simulink model "register"  (R2024a)
settings: Solver=FixedStepDiscrete  StartTime=1  StopTime=inf  RelTol=1e-3  EnableMultiTasking=on
libraries: simulink_extras x5
settings Model: Creator=nunkesser  LastModifiedBy=nunkesser
settings SolverCC: AlgebraicLoopSolver=TrustRegion
settings DataIOCC: LimitDataPoints=on  SaveFormat=Array  ReturnWorkspaceOutputs=off
settings OptimizationCC: LifeSpan=inf
settings DebuggingCC: SolverPrmCheckMsg=warning  UnconnectedInputMsg=warning  UnconnectedOutputMsg=warning  UnconnectedLineMsg=warning  SFUnexpectedBacktrackingDiag=warning  SFNoUnconditionalDefaultTransitionDiag=warning  SFExecutionAtInitializationDiag=none  ArithmeticOperatorsInVariantConditions=warning
settings HardwareCC: ProdBitPerPointer=32  ProdBitPerSizeT=32  ProdBitPerPtrDiffT=32  ProdLargestAtomicFloat=None  ProdIntDivRoundTo=Undefined  ProdEndianess=Unspecified  ProdWordSize=32  ProdHWDeviceType=32-bit Generic
settings ModelReferenceCC: PropagateSignalLabelsOutOfModel=off
settings SFSimCC: SimUseLocalCustomCode=off  CustomCodeUndefinedFunction=UseInterfaceOnly
settings RTWCC: RTWUseLocalCustomCode=off  GPUComputeCapability=3.5
settings CodeAppCC: StateflowObjectComments=on
settings GRTTargetCC: TargetLangStandard=C89/C90 (ANSI)
settings ConfigComp: CovMetricSettings=dw  CovSaveCumulativeToWorkspaceVar=on  CovSaveSingleToWorkspaceVar=on  CovExternalEMLEnable=off  CovSFcnEnable=off
settings ConfigurationSet: Description=SimMechanics 2G

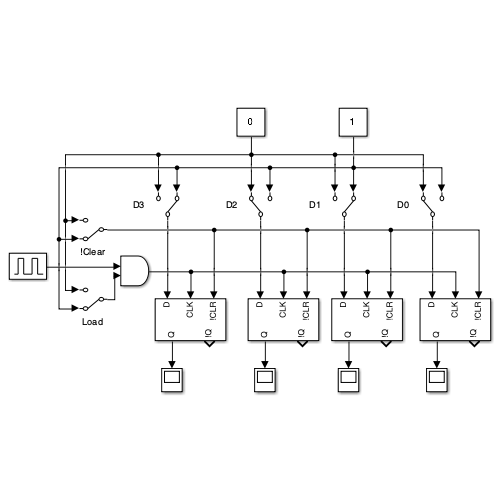
[thumbnail: Simulink's stored preview of the top-level diagram]
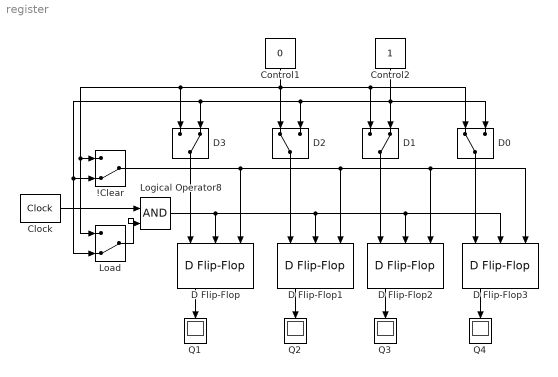
== system register ==
  !Clear : ManualSwitch  CurrentSetting=0
  Clock : simulink_extras/Flip Flops/Clock  period=2
  Control1 : Constant  Value=0  OutDataTypeStr=boolean
  Control2 : Constant  OutDataTypeStr=boolean
  D Flip-Flop{,1..3} (4 alike) : simulink_extras/Flip Flops/D Flip-Flop
  D0 : ManualSwitch
  D1 : ManualSwitch  CurrentSetting=0
  D2 : ManualSwitch
  D3 : ManualSwitch  CurrentSetting=0
  Load : ManualSwitch  CurrentSetting=0
  Logical Operator8 : Logic  IconShape=distinctive  AllPortsSameDT=off  OutDataTypeStr=boolean
  Q{1..4} (4 alike) : Display
  wires:
  Control1/1 -> D3/1, Load/1, !Clear/1, D2/1, D1/1, D0/1
  Control2/1 -> D2/2, D3/2, Load/2, !Clear/2, D1/2, D0/2
  !Clear/1 -> D Flip-Flop/3, D Flip-Flop1/3, D Flip-Flop2/3, D Flip-Flop3/3
  D Flip-Flop/1 -> Q1/1
  D Flip-Flop1/1 -> Q2/1
  D Flip-Flop2/1 -> Q3/1
  D Flip-Flop3/1 -> Q4/1
  D0/1 -> D Flip-Flop3/1
  D1/1 -> D Flip-Flop2/1
  D2/1 -> D Flip-Flop1/1
  D3/1 -> D Flip-Flop/1
  Clock/1 -> Logical Operator8/1
  Load/1 -> Logical Operator8/2
  Logical Operator8/1 -> D Flip-Flop/2, D Flip-Flop1/2, D Flip-Flop3/2, D Flip-Flop2/2
